simulink model "logo_monitoring_exec"  (Simulink 3.00)
libraries: execlib x5

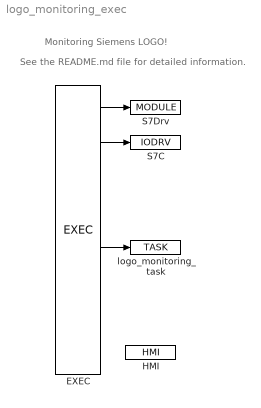
== system logo_monitoring_exec ==
  note: Monitoring Siemens LOGO!
  note: See the README.md file for detailed information.
  EXEC : execlib/EXEC  target=Generic target device  tick=0.01  ntick0=10  ntick1=50  ntick2=100  ntick3=1200  pri0=5  pri1=9  pri2=13  pri3=18
  HMI : execlib/HMI  IncludeHMI=on  HmiDir=hmi  SourceDir=hmisrc  GenerateWebWatch=on  GenerateRexHMI=on  RedirectToHMI=off  Compression=off
  S7C : execlib/IODRV  module=S7Drv  classname=S7cDrv  cfgname=logo_iocfg.rio  factor=5  stack=10240  pri=3  timer=off
  S7Drv : execlib/MODULE
  logo_monitoring_task : execlib/TASK  factor=1  start=0  stop=1  stack=10240  MDLOPEN=on
  wires:
  EXEC/1 -> S7Drv/1
  EXEC/2 -> S7C/1
  EXEC/5 -> logo_monitoring_task/1
